simulink model "Original"  (R2019a)
settings: Solver=VariableStepAuto  StartTime=0.0  StopTime=5  RelTol=1e-3
values from neighbouring files (symbols this model uses):
  g = 9.81    [Data.m]    (also in func.m; myTransitionFcn.m)
  m = 0.1    [Data.m]    (also in myTransitionFcn.m)
  r = 0.1    [Data.m]    (also in func.m; myTransitionFcn.m)
  R = 1    [Data.m]    (also in func.m; myTransitionFcn.m)
libraries: simulink x1
settings Model: Creator=Dell  LastModifiedBy=Dell

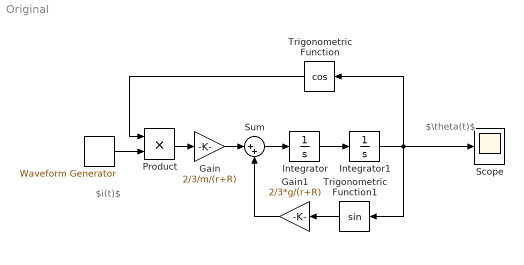
== system Original ==
  note: $i(t)$
  note: $\theta(t)$
  " " : simulink/Sources/Waveform Generator  OutMin=[]  OutMax=[]  OutDataTypeStr=double  SelectedSignal=1  Signals=step()  BlockNames=MultiportSwitch_8c7b78d12e5b405  SampleTime=0.1
      settings: SourceProductName=Simulink
  Gain : Gain  Gain=2/3/m/(r+R)
  Gain1 : Gain  Gain=2/3*g/(r+R)
  Integrator : Integrator
  Integrator1 : Integrator
  Product : Product
  Scope : Scope
  Sum : Sum  Inputs=|++
  Trigonometric Function : Trigonometry  Operator=cos
  Trigonometric Function1 : Trigonometry
  wires:
  Integrator1/1 -> Trigonometric Function1/1, Scope/1, Trigonometric Function/1
  Integrator/1 -> Integrator1/1
  Trigonometric Function/1 -> Product/1
  Gain1/1 -> Sum/2
  Product/1 -> Gain/1
  Trigonometric Function1/1 -> Gain1/1
  " "/1 -> Product/2
  Gain/1 -> Sum/1
  Sum/1 -> Integrator/1
